simulink model "heli_sim"  (Simulink 7.7)
settings: Solver=ode4  SolverMode=SingleTasking  StartTime=0.0  StopTime=30  FixedStep=1/250  RelTol=1e-3
PostLoadFcn:
  | if exist('helicopter_sim.mat', 'file')
  |     load helicopter_sim.mat;
  | end
undefined symbols (not defined in the file or in its folder): alpha_IERA_IELA_IELA, in_cmd_final_value, in_CMD_ini, in_cmd_step_time, in_d_ini, in_omega_MR, in_omega_TR, in_outside_air_temp, in_pressure_altitude, in_xc_EOM_ini, R_IERA_RA_RA
libraries: simulink x4, UAVdesign_net x3
settings Model: Creator=Emanuel  LastModifiedBy=Emanuel  ExtModeLogAll=off
settings DataIOCC: LimitDataPoints=off  SaveFormat=StructureWithTime  SaveOutput=off  SignalLogging=off  SaveTime=off
settings OptimizationCC: InlineParams=on  SimCompilerOptimization=On
settings DebuggingCC: StrictBusMsg=Warning
settings HardwareCC: ProdIntDivRoundTo=Zero  ProdEndianess=LittleEndian  ProdHWDeviceType=Generic->32-bit x86 compatible
settings SFSimCC: SimParseCustomCode=off
settings RTWCC: RTWCompilerOptimization=On

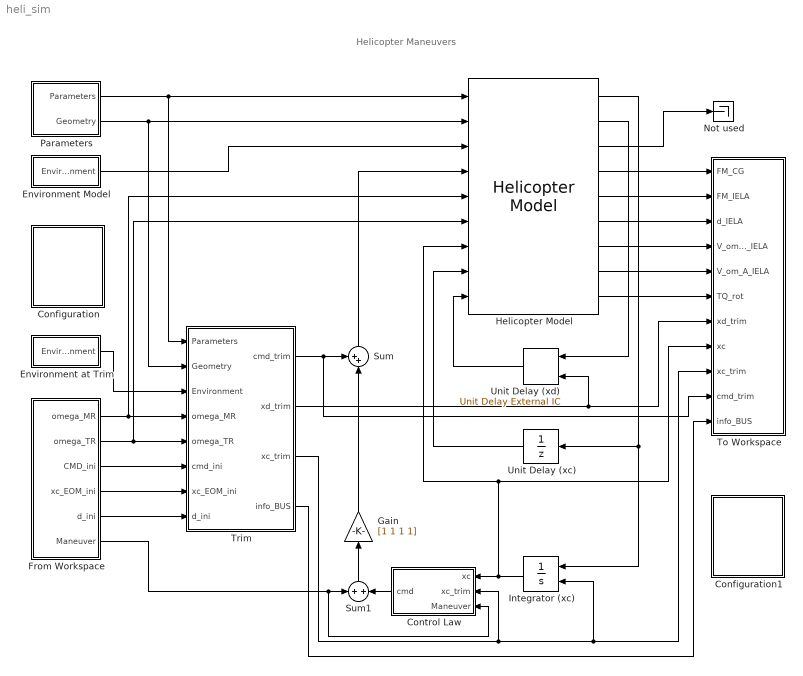
== system heli_sim ==
  note: Helicopter Maneuvers
  Configuration : Subsystem
      settings: OpenFcn=gui_HelicopterSim;
      mask Display: disp('Double-click\nto configure\nthe\nsimulation')
  Configuration1 : Subsystem
      settings: OpenFcn=graphs_Helicopter_sim;
      mask Display: disp('Double-click\nto display\nthe\ngraphs')
  Control Law : Subsystem
  Environment at Trim : Subsystem
  Environment Model : Subsystem
  From Workspace : Subsystem
  Gain : Gain  Gain=[1 1 1 1]
  Helicopter Model : UAVdesign_net/Vehicle Models/Helicopter Model  SystemSampleTime=-1
  Integrator (xc) : Integrator  InitialConditionSource=external  LimitOutput=on  UpperSaturationLimit="[1 1 1 1  1 1 1 1 100 100 100 inf inf inf pi/4 pi/4 pi/4 inf inf inf pi/4 pi/4 pi/4 pi/4 pi/4 pi/4]"  LowerSaturationLimit="-[1 1 1 1  1 1 1 1 100 100 100 inf inf inf pi/4 pi/4 pi/4 inf inf inf pi/4 pi/4 pi/4 pi/4 pi/4 pi/4]"
  Not used : Terminator
  Parameters : Subsystem
      mask init:
      | set_param(gcb, 'LinkStatus', 'none');
      settings: OpenFcn=gui_HelicopterParameters( 'Block', [get_param(gcb, 'Parent') '/' get_param(gcb, 'Name')]);
      mask Display:
      | port_label('output', 1, 'Parameters')
      | port_label('output', 2, 'Geometry')
  Sum : Sum  Inputs=++|
  Sum1 : Sum  Inputs=+|+
  To Workspace : Subsystem
  Trim : Subsystem
  Unit Delay (xc) : UnitDelay  X0=zeros(26,1)  SampleTime=1/250
  Unit Delay (xd) : simulink/Additional Math & Discrete/Additional Discrete/Unit Delay External IC  SystemSampleTime=-1  tsamp=1/250
  wires:
  Parameters/2(Geometry) -> Helicopter Model/2, Trim/2(Geometry)
  Parameters/1(Parameters) -> Helicopter Model/1, Trim/1(Parameters)
  Environment Model/1(Environment) -> Helicopter Model/3
  Unit Delay (xd)/1 -> Helicopter Model/9
  Helicopter Model/2 -> Unit Delay (xd)/1
  Trim/2(xd_trim) -> Unit Delay (xd)/2, To Workspace/7(xd_trim)
  Helicopter Model/1 -> Unit Delay (xc)/1, Integrator (xc)/1
  Unit Delay (xc)/1 -> Helicopter Model/8
  From Workspace/3(CMD_ini) -> Trim/6(cmd_ini)
  From Workspace/4(xc_EOM_ini) -> Trim/7(xc_EOM_ini)
  From Workspace/5(d_ini) -> Trim/8(d_ini)
  Integrator (xc)/1 -> Control Law/1(xc), Helicopter Model/7, To Workspace/8(xc)
  Trim/1(cmd_trim) -> Sum/1, To Workspace/10(cmd_trim)
  Sum/1 -> Helicopter Model/4
  Environment at Trim/1(Environment) -> Trim/3(Environment)
  From Workspace/2(omega_TR) -> Trim/5(omega_TR), Helicopter Model/6
  From Workspace/1(omega_MR) -> Trim/4(omega_MR), Helicopter Model/5
  Helicopter Model/3 -> Not used/1
  Helicopter Model/4 -> To Workspace/1(FM_CG)
  Helicopter Model/5 -> To Workspace/2(FM_IELA)
  Helicopter Model/6 -> To Workspace/3(d_IELA)
  Helicopter Model/7 -> To Workspace/4(V_om_W_IELA)
  Trim/4(info_BUS) -> To Workspace/11(info_BUS)
  Control Law/1(cmd) -> Sum1/2
  Trim/3(xc_trim) -> Control Law/2(xc_trim), Integrator (xc)/2, To Workspace/9(xc_trim)
  From Workspace/6(Maneuver) -> Sum1/1, Control Law/3(Maneuver)
  Helicopter Model/8 -> To Workspace/5(V_om_A_IELA)
  Helicopter Model/9 -> To Workspace/6(TQ_rot)
  Gain/1 -> Sum/2
  Sum1/1 -> Gain/1

== system heli_sim/Configuration ==

== system heli_sim/Configuration1 ==

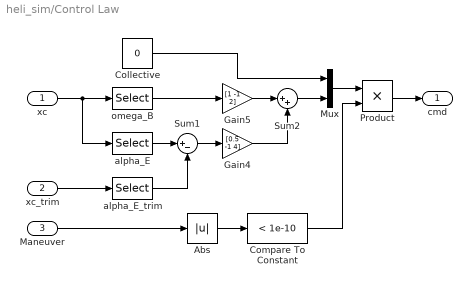
== system heli_sim/Control Law ==
  xc : Inport
  xc_trim : Inport  Port=2
  Maneuver : Inport  Port=3
  Abs : Abs
  Collective : Constant  Value=0
  Compare To Constant : simulink/Logic and Bit Operations/Compare To Constant  SystemSampleTime=-1  relop=<  const=1e-10  LogicOutDataTypeMode=boolean  ZeroCross=off
  Gain4 : Gain  Gain=[0.5 -1 4]
  Gain5 : Gain  Gain=[1 -1 2]
  Mux : Mux  Inputs=2
  Product : Product  RndMeth=Zero
  Sum1 : Sum  Inputs=|+-
  Sum2 : Sum  Inputs=|++
  alpha_E : Selector  InputPortWidth=26  IndexOptions=Index vector (dialog)  Indices=[18:20]  OutputSizes=1
  alpha_E_trim : Selector  InputPortWidth=26  IndexOptions=Index vector (dialog)  Indices=[18:20]  OutputSizes=1
  omega_B : Selector  InputPortWidth=26  IndexOptions=Index vector (dialog)  Indices=[15:17]  OutputSizes=1
  cmd : Outport
  wires:
  alpha_E_trim/1 -> Sum1/2
  alpha_E/1 -> Sum1/1
  Sum1/1 -> Gain4/1
  omega_B/1 -> Gain5/1
  xc/1 -> omega_B/1, alpha_E/1
  xc_trim/1 -> alpha_E_trim/1
  Gain5/1 -> Sum2/1
  Gain4/1 -> Sum2/2
  Sum2/1 -> Mux/2
  Collective/1 -> Mux/1
  Maneuver/1 -> Abs/1
  Mux/1 -> Product/1
  Product/1 -> cmd/1
  Compare To Constant/1 -> Product/2
  Abs/1 -> Compare To Constant/1

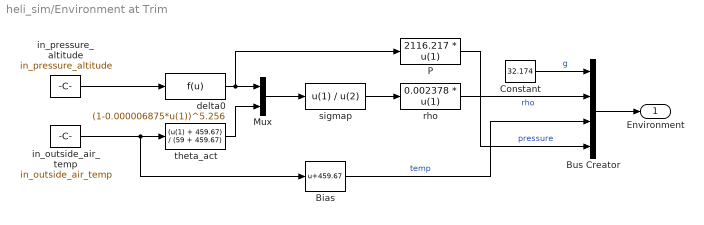
== system heli_sim/Environment at Trim ==
  Bias : Bias  Bias=459.67
  Bus Creator : BusCreator  OutDataTypeStr=Bus: Environment  NonVirtualBus=on
  Constant : Constant  Value=32.174
  Mux : Mux  Inputs=2
  P : Fcn  Expr=2116.217 * u(1)
  delta0 : Fcn  Expr=(1-0.000006875*u(1))^5.256
  in_outside_air_temp : Constant  Value=in_outside_air_temp
  in_pressure_altitude : Constant  Value=in_pressure_altitude
  rho : Fcn  Expr=0.002378 * u(1)
  sigmap : Fcn  Expr=u(1) / u(2)
  theta_act : Fcn  Expr=(u(1) + 459.67) / (59 + 459.67)
  Environment : Outport  OutDataTypeStr=Bus: Environment
  wires:
  sigmap/1 -> rho/1
  theta_act/1 -> Mux/2
  Mux/1 -> sigmap/1
  in_outside_air_temp/1 -> Bias/1, theta_act/1
  delta0/1 -> P/1, Mux/1
  in_pressure_altitude/1 -> delta0/1
  Bus Creator/1 -> Environment/1
  Constant/1 -> Bus Creator/1  "g"
  rho/1 -> Bus Creator/2  "rho"
  Bias/1 -> Bus Creator/3  "temp"
  P/1 -> Bus Creator/4  "pressure"

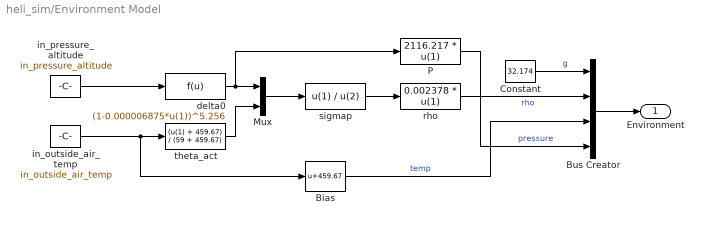
== system heli_sim/Environment Model ==
  Bias : Bias  Bias=459.67
  Bus Creator : BusCreator  OutDataTypeStr=Bus: Environment  NonVirtualBus=on
  Constant : Constant  Value=32.174
  Mux : Mux  Inputs=2
  P : Fcn  Expr=2116.217 * u(1)
  delta0 : Fcn  Expr=(1-0.000006875*u(1))^5.256
  in_outside_air_temp : Constant  Value=in_outside_air_temp
  in_pressure_altitude : Constant  Value=in_pressure_altitude
  rho : Fcn  Expr=0.002378 * u(1)
  sigmap : Fcn  Expr=u(1) / u(2)
  theta_act : Fcn  Expr=(u(1) + 459.67) / (59 + 459.67)
  Environment : Outport  OutDataTypeStr=Bus: Environment
  wires:
  P/1 -> Bus Creator/4  "pressure"
  Bias/1 -> Bus Creator/3  "temp"
  rho/1 -> Bus Creator/2  "rho"
  Constant/1 -> Bus Creator/1  "g"
  Bus Creator/1 -> Environment/1
  in_pressure_altitude/1 -> delta0/1
  delta0/1 -> Mux/1, P/1
  in_outside_air_temp/1 -> theta_act/1, Bias/1
  Mux/1 -> sigmap/1
  theta_act/1 -> Mux/2
  sigmap/1 -> rho/1

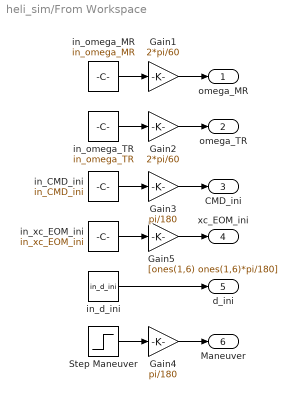
== system heli_sim/From Workspace ==
  Gain1 : Gain  Gain=2*pi/60
  Gain2 : Gain  Gain=2*pi/60
  Gain3 : Gain  Gain=pi/180
  Gain4 : Gain  Gain=pi/180
  Gain5 : Gain  Gain=[ones(1,6) ones(1,6)*pi/180]
  Step Maneuver : Step  Time=in_cmd_step_time  Before=[0 0 0 0]  After=in_cmd_final_value  SampleTime=0
  in_CMD_ini : Constant  Value=in_CMD_ini
  in_d_ini : Constant  Value=in_d_ini
  in_omega_MR : Constant  Value=in_omega_MR
  in_omega_TR : Constant  Value=in_omega_TR
  in_xc_EOM_ini : Constant  Value=in_xc_EOM_ini
  omega_MR : Outport
  omega_TR : Outport  Port=2
  CMD_ini : Outport  Port=3
  xc_EOM_ini : Outport  Port=4
  d_ini : Outport  Port=5
  Maneuver : Outport  Port=6
  wires:
  in_omega_MR/1 -> Gain1/1
  in_omega_TR/1 -> Gain2/1
  in_CMD_ini/1 -> Gain3/1
  in_xc_EOM_ini/1 -> Gain5/1
  in_d_ini/1 -> d_ini/1
  Gain4/1 -> Maneuver/1
  Step Maneuver/1 -> Gain4/1
  Gain1/1 -> omega_MR/1
  Gain2/1 -> omega_TR/1
  Gain3/1 -> CMD_ini/1
  Gain5/1 -> xc_EOM_ini/1

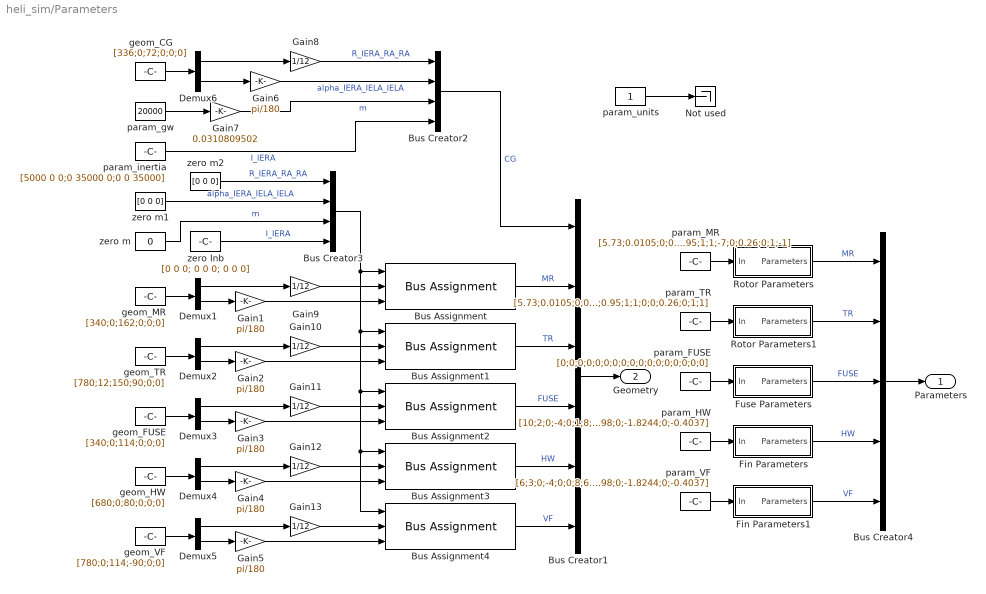
== system heli_sim/Parameters ==
  Bus Assignment{,1..4} (5 alike) : BusAssignment  AssignedSignals=R_IERA_RA_RA,alpha_IERA_IELA_IELA
  Bus Creator1 : BusCreator  Inputs=6
  Bus Creator2 : BusCreator  OutDataTypeStr=Bus: GeometryParameters
  Bus Creator3 : BusCreator  OutDataTypeStr=Bus: GeometryParameters
  Bus Creator4 : BusCreator  Inputs=5
  Demux{1..6} (6 alike) : Demux  Outputs=2
  Fin Parameters : Subsystem
  Fin Parameters1 : Subsystem
  Fuse Parameters : Subsystem
  Gain{1..6} (6 alike) : Gain  Gain=pi/180
  Gain{8..13} (6 alike) : Gain  Gain=1/12
  Gain7 : Gain  Gain=0.0310809502
  Not used : Terminator
  Rotor Parameters : Subsystem
  Rotor Parameters1 : Subsystem
  geom_CG : Constant  Value=[336;0;72;0;0;0]
  geom_FUSE : Constant  Value=[340;0;114;0;0;0]
  geom_HW : Constant  Value=[680;0;80;0;0;0]
  geom_MR : Constant  Value=[340;0;162;0;0;0]
  geom_TR : Constant  Value=[780;12;150;90;0;0]
  geom_VF : Constant  Value=[780;0;114;-90;0;0]
  param_FUSE : Constant  Value=[0;0;0;0;0;0;0;0;0;0;0;0;0;0;0;0;0]
  param_HW : Constant  Value=[10;2;0;-4;0;1;8;6.13;0.9682;1.8898;0;-1.8244;0;-0.4037]
  param_MR : Constant  Value=[5.73;0.0105;0;0.01325;0;-15;0;0;7;30;2.5;0.95;1;1;-7;0;0.26;0;1;-1]
  param_TR : Constant  Value=[5.73;0.0105;0;0.01325;0;-45;0;0;4;6.5;1.25;0.95;1;1;0;0;0.26;0;1;1]
  param_VF : Constant  Value=[6;3;0;-4;0;0;8;6.1311;0.9682;1.8898;0;-1.8244;0;-0.4037]
  param_gw : Constant  Value=20000
  param_inertia : Constant  Value=[5000 0 0;0 35000 0;0 0 35000]
  param_units : Constant
  zero Inb : Constant  Value=[0 0 0; 0 0 0; 0 0 0]
  zero m : Constant  Value=0
  zero m1 : Constant  Value=[0 0 0]
  zero m2 : Constant  Value=[0 0 0]
  Parameters : Outport
  Geometry : Outport  Port=2
  wires:
  Bus Creator2/1 -> Bus Creator1/1  "CG"
  Bus Assignment1/1 -> Bus Creator1/3  "TR"
  Bus Assignment2/1 -> Bus Creator1/4  "FUSE"
  Bus Assignment3/1 -> Bus Creator1/5  "HW"
  Bus Assignment4/1 -> Bus Creator1/6  "VF"
  Bus Creator1/1 -> Geometry/1
  Demux6/1 -> Gain8/1
  Demux6/2 -> Gain6/1
  param_gw/1 -> Gain7/1
  param_inertia/1 -> Bus Creator2/4  "I_IERA"
  Bus Assignment/1 -> Bus Creator1/2  "MR"
  Demux1/1 -> Gain9/1
  Demux1/2 -> Gain1/1
  geom_MR/1 -> Demux1/1
  Demux2/1 -> Gain10/1
  Demux2/2 -> Gain2/1
  geom_TR/1 -> Demux2/1
  Demux3/1 -> Gain11/1
  Demux3/2 -> Gain3/1
  geom_FUSE/1 -> Demux3/1
  Demux4/1 -> Gain12/1
  Demux4/2 -> Gain4/1
  geom_HW/1 -> Demux4/1
  Demux5/1 -> Gain13/1
  Demux5/2 -> Gain5/1
  geom_VF/1 -> Demux5/1
  geom_CG/1 -> Demux6/1
  Bus Creator3/1 -> Bus Assignment/1, Bus Assignment1/1, Bus Assignment2/1, Bus Assignment4/1, Bus Assignment3/1
  zero m/1 -> Bus Creator3/3  "m"
  zero m1/1 -> Bus Creator3/2  "alpha_IERA_IELA_IELA"
  zero Inb/1 -> Bus Creator3/4  "I_IERA"
  zero m2/1 -> Bus Creator3/1  "R_IERA_RA_RA"
  Bus Creator4/1 -> Parameters/1
  Rotor Parameters/1(Parameters) -> Bus Creator4/1  "MR"
  param_MR/1 -> Rotor Parameters/1(In)
  Rotor Parameters1/1(Parameters) -> Bus Creator4/2  "TR"
  param_TR/1 -> Rotor Parameters1/1(In)
  param_FUSE/1 -> Fuse Parameters/1(In)
  Fuse Parameters/1(Parameters) -> Bus Creator4/3  "FUSE"
  param_VF/1 -> Fin Parameters1/1(In)
  Fin Parameters1/1(Parameters) -> Bus Creator4/5  "VF"
  Fin Parameters/1(Parameters) -> Bus Creator4/4  "HW"
  param_HW/1 -> Fin Parameters/1(In)
  Gain1/1 -> Bus Assignment/3
  Gain2/1 -> Bus Assignment1/3
  Gain3/1 -> Bus Assignment2/3
  Gain4/1 -> Bus Assignment3/3
  Gain5/1 -> Bus Assignment4/3
  Gain6/1 -> Bus Creator2/2  "alpha_IERA_IELA_IELA"
  Gain7/1 -> Bus Creator2/3  "m"
  Gain8/1 -> Bus Creator2/1  "R_IERA_RA_RA"
  Gain9/1 -> Bus Assignment/2
  Gain10/1 -> Bus Assignment1/2
  Gain11/1 -> Bus Assignment2/2
  Gain12/1 -> Bus Assignment3/2
  Gain13/1 -> Bus Assignment4/2
  param_units/1 -> Not used/1

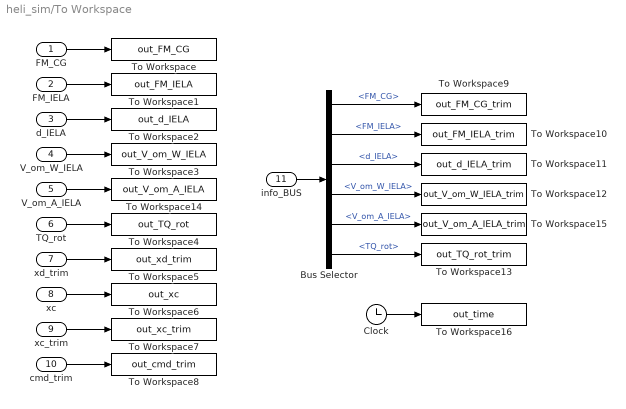
== system heli_sim/To Workspace ==
  FM_CG : Inport
  FM_IELA : Inport  Port=2
  d_IELA : Inport  Port=3
  V_om_W_IELA : Inport  Port=4
  V_om_A_IELA : Inport  Port=5
  TQ_rot : Inport  Port=6
  xd_trim : Inport  Port=7
  xc : Inport  Port=8
  xc_trim : Inport  Port=9
  cmd_trim : Inport  Port=10
  info_BUS : Inport  Port=11
  Bus Selector : BusSelector  OutputSignals=FM_CG,FM_IELA,d_IELA,V_om_W_IELA,V_om_A_IELA,TQ_rot
  Clock : Clock
  To Workspace : ToWorkspace  VariableName=out_FM_CG  SampleTime=-1  SaveFormat=Array
  To Workspace1 : ToWorkspace  VariableName=out_FM_IELA  SampleTime=-1  SaveFormat=Array
  To Workspace10 : ToWorkspace  VariableName=out_FM_IELA_trim  SampleTime=-1  SaveFormat=Array
      settings: MaxDataPoints=1
  To Workspace11 : ToWorkspace  VariableName=out_d_IELA_trim  SampleTime=-1  SaveFormat=Array
      settings: MaxDataPoints=1
  To Workspace12 : ToWorkspace  VariableName=out_V_om_W_IELA_trim  SampleTime=-1  SaveFormat=Array
      settings: MaxDataPoints=1
  To Workspace13 : ToWorkspace  VariableName=out_TQ_rot_trim  SampleTime=-1  SaveFormat=Array
      settings: MaxDataPoints=1
  To Workspace14 : ToWorkspace  VariableName=out_V_om_A_IELA  SampleTime=-1  SaveFormat=Array
  To Workspace15 : ToWorkspace  VariableName=out_V_om_A_IELA_trim  SampleTime=-1  SaveFormat=Array
      settings: MaxDataPoints=1
  To Workspace16 : ToWorkspace  VariableName=out_time  SampleTime=-1  SaveFormat=Array
  To Workspace2 : ToWorkspace  VariableName=out_d_IELA  SampleTime=-1  SaveFormat=Array
  To Workspace3 : ToWorkspace  VariableName=out_V_om_W_IELA  SampleTime=-1  SaveFormat=Array
  To Workspace4 : ToWorkspace  VariableName=out_TQ_rot  SampleTime=-1  SaveFormat=Array
  To Workspace5 : ToWorkspace  VariableName=out_xd_trim  SampleTime=-1  SaveFormat=Array
      settings: MaxDataPoints=1
  To Workspace6 : ToWorkspace  VariableName=out_xc  SampleTime=-1  SaveFormat=Array
  To Workspace7 : ToWorkspace  VariableName=out_xc_trim  SampleTime=-1  SaveFormat=Array
      settings: MaxDataPoints=1
  To Workspace8 : ToWorkspace  VariableName=out_cmd_trim  SampleTime=-1  SaveFormat=Array
      settings: MaxDataPoints=1
  To Workspace9 : ToWorkspace  VariableName=out_FM_CG_trim  SampleTime=-1  SaveFormat=Array
      settings: MaxDataPoints=1
  wires:
  FM_CG/1 -> To Workspace/1
  FM_IELA/1 -> To Workspace1/1
  d_IELA/1 -> To Workspace2/1
  V_om_W_IELA/1 -> To Workspace3/1
  TQ_rot/1 -> To Workspace4/1
  xd_trim/1 -> To Workspace5/1
  xc/1 -> To Workspace6/1
  xc_trim/1 -> To Workspace7/1
  cmd_trim/1 -> To Workspace8/1
  info_BUS/1 -> Bus Selector/1
  Bus Selector/1 -> To Workspace9/1  "<FM_CG>"
  Bus Selector/2 -> To Workspace10/1  "<FM_IELA>"
  Bus Selector/3 -> To Workspace11/1  "<d_IELA>"
  Bus Selector/4 -> To Workspace12/1  "<V_om_W_IELA>"
  Bus Selector/6 -> To Workspace13/1  "<TQ_rot>"
  V_om_A_IELA/1 -> To Workspace14/1
  Bus Selector/5 -> To Workspace15/1  "<V_om_A_IELA>"
  Clock/1 -> To Workspace16/1

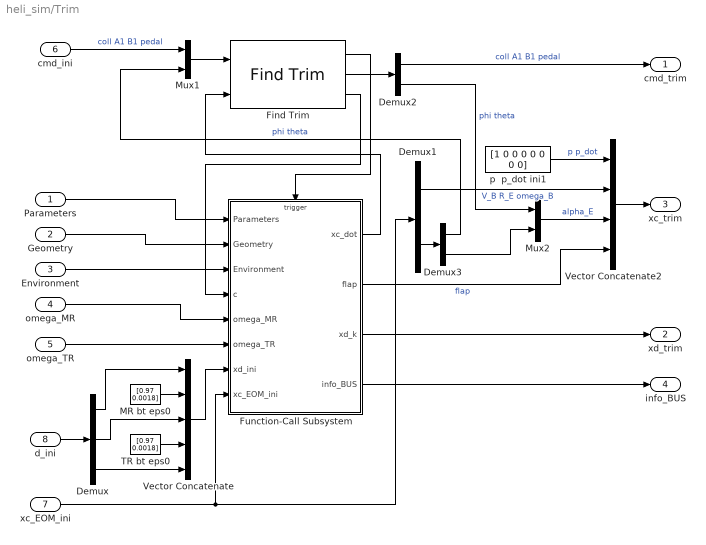
== system heli_sim/Trim ==
  Parameters : Inport
  Geometry : Inport  Port=2
  Environment : Inport  Port=3
  omega_MR : Inport  Port=4
  omega_TR : Inport  Port=5
  cmd_ini : Inport  Port=6
  xc_EOM_ini : Inport  Port=7
  d_ini : Inport  Port=8
  Demux : Demux  Outputs=[3 3 9]
  Demux1 : Demux  Outputs=[9 3]
  Demux2 : Demux  Outputs=[4 2]
  Demux3 : Demux  Outputs=[2 1]
  Find Trim : UAVdesign_net/Utilities/Numeric Perturbation/Find Trim  NumFInputs=6  NumFOutputs=6  RunOnce=on  SampleTime=-1
  Function-Call Subsystem : Subsystem  TreatAsAtomicUnit=on
  MR bt eps0 : Constant  Value=[0.97 0.0018]
  Mux1 : Mux  Inputs=2
  Mux2 : Mux  Inputs=2
  TR bt eps0 : Constant  Value=[0.97 0.0018]
  Vector Concatenate : Concatenate  NumInputs=5  Mode=Vector
  Vector Concatenate2 : Concatenate  NumInputs=4  Mode=Vector
  p  p_dot ini1 : Constant  Value="[1 0 0 0  0 0 0 0]"
  cmd_trim : Outport
  xd_trim : Outport  Port=2
  xc_trim : Outport  Port=3
  info_BUS : Outport  Port=4
  wires:
  Geometry/1 -> Function-Call Subsystem/2(Geometry)
  Parameters/1 -> Function-Call Subsystem/1(Parameters)
  omega_MR/1 -> Function-Call Subsystem/5(omega_MR)
  xc_EOM_ini/1 -> Function-Call Subsystem/8(xc_EOM_ini), Demux1/1
  omega_TR/1 -> Function-Call Subsystem/6(omega_TR)
  Find Trim/3 -> Function-Call Subsystem/4(c)
  Function-Call Subsystem/1(xc_dot) -> Find Trim/2
  Find Trim/1 -> Function-Call Subsystem/Trigger
  Function-Call Subsystem/3(xd_k) -> xd_trim/1
  d_ini/1 -> Demux/1
  Demux/1 -> Vector Concatenate/1
  MR bt eps0/1 -> Vector Concatenate/2
  Demux/2 -> Vector Concatenate/3
  TR bt eps0/1 -> Vector Concatenate/4
  Demux/3 -> Vector Concatenate/5
  Vector Concatenate/1 -> Function-Call Subsystem/7(xd_ini)
  Find Trim/2 -> Demux2/1
  Demux2/1 -> cmd_trim/1  "coll A1 B1 pedal"
  Mux1/1 -> Find Trim/1
  cmd_ini/1 -> Mux1/1  "coll A1 B1 pedal"
  Vector Concatenate2/1 -> xc_trim/1
  p  p_dot ini1/1 -> Vector Concatenate2/1  "p p_dot"
  Demux1/1 -> Vector Concatenate2/2  "V_B R_E omega_B"
  Mux2/1 -> Vector Concatenate2/3  "alpha_E"
  Function-Call Subsystem/2(flap) -> Vector Concatenate2/4  "flap"
  Demux3/2 -> Mux2/2
  Demux1/2 -> Demux3/1
  Demux2/2 -> Mux2/1  "phi theta"
  Demux3/1 -> Mux1/2  "phi theta"
  Environment/1 -> Function-Call Subsystem/3(Environment)
  Function-Call Subsystem/4(info_BUS) -> info_BUS/1

== system heli_sim/Parameters/Fin Parameters ==
  In : Inport
  Bus Creator : BusCreator  Inputs=14  OutDataTypeStr=Bus: FinParameters  NonVirtualBus=on
  Demux : Demux  Outputs=14
  Gain{,1..3} (4 alike) : Gain  Gain=pi/180
  Parameters : Outport  OutDataTypeStr=Bus: FinParameters
  wires:
  In/1 -> Demux/1
  Bus Creator/1 -> Parameters/1
  Demux/1 -> Bus Creator/1  "span"
  Demux/2 -> Bus Creator/2  "chord"
  Demux/3 -> Gain2/1
  Gain2/1 -> Bus Creator/3  "dihedral"
  Demux/4 -> Gain/1
  Gain/1 -> Bus Creator/4  "incid"
  Gain1/1 -> Bus Creator/5  "sweep"
  Demux/5 -> Gain1/1
  Demux/6 -> Bus Creator/6  "taper"
  Demux/7 -> Gain3/1
  Gain3/1 -> Bus Creator/7  "stall"
  Demux/8 -> Bus Creator/8  "a0"
  Demux/9 -> Bus Creator/9  "a1s2"
  Demux/10 -> Bus Creator/10  "cd0"
  Demux/11 -> Bus Creator/11  "cd1s1"
  Demux/12 -> Bus Creator/12  "cd2c1"
  Demux/13 -> Bus Creator/13  "cm0"
  Demux/14 -> Bus Creator/14  "cm1s1"

== system heli_sim/Parameters/Fin Parameters1 ==
  In : Inport
  Bus Creator : BusCreator  Inputs=14  OutDataTypeStr=Bus: FinParameters  NonVirtualBus=on
  Demux : Demux  Outputs=14
  Gain{,1..3} (4 alike) : Gain  Gain=pi/180
  Parameters : Outport  OutDataTypeStr=Bus: FinParameters
  wires:
  Demux/14 -> Bus Creator/14  "cm1s1"
  Demux/13 -> Bus Creator/13  "cm0"
  Demux/12 -> Bus Creator/12  "cd2c1"
  Demux/11 -> Bus Creator/11  "cd1s1"
  Demux/10 -> Bus Creator/10  "cd0"
  Demux/9 -> Bus Creator/9  "a1s2"
  Demux/8 -> Bus Creator/8  "a0"
  Gain3/1 -> Bus Creator/7  "stall"
  Demux/7 -> Gain3/1
  Demux/6 -> Bus Creator/6  "taper"
  Demux/5 -> Gain1/1
  Gain1/1 -> Bus Creator/5  "sweep"
  Gain/1 -> Bus Creator/4  "incid"
  Demux/4 -> Gain/1
  Gain2/1 -> Bus Creator/3  "dihedral"
  Demux/3 -> Gain2/1
  Demux/2 -> Bus Creator/2  "chord"
  Demux/1 -> Bus Creator/1  "span"
  Bus Creator/1 -> Parameters/1
  In/1 -> Demux/1

== system heli_sim/Parameters/Fuse Parameters ==
  In : Inport
  Bus Creator : BusCreator  Inputs=7  OutDataTypeStr=Bus: FuselageParameters  NonVirtualBus=on
  Demux : Demux  Outputs=17
  Vector Concatenate{,1..4} (5 alike) : Concatenate  NumInputs=3  Mode=Vector
  Parameters : Outport  OutDataTypeStr=Bus: FuselageParameters
  wires:
  Demux/1 -> Bus Creator/1  "carea"
  Bus Creator/1 -> Parameters/1
  In/1 -> Demux/1
  Demux/2 -> Bus Creator/2  "clen"
  Demux/3 -> Vector Concatenate/1
  Demux/4 -> Vector Concatenate/2
  Demux/5 -> Vector Concatenate/3
  Vector Concatenate/1 -> Bus Creator/3  "cx"
  Demux/6 -> Vector Concatenate1/1
  Demux/7 -> Vector Concatenate1/2
  Demux/8 -> Vector Concatenate1/3
  Vector Concatenate1/1 -> Bus Creator/4  "cy"
  Demux/9 -> Vector Concatenate2/1
  Demux/10 -> Vector Concatenate2/2
  Demux/11 -> Vector Concatenate2/3
  Vector Concatenate2/1 -> Bus Creator/5  "cz"
  Demux/12 -> Vector Concatenate3/1
  Demux/13 -> Vector Concatenate3/2
  Demux/14 -> Vector Concatenate3/3
  Demux/15 -> Vector Concatenate4/1
  Demux/16 -> Vector Concatenate4/2
  Demux/17 -> Vector Concatenate4/3
  Vector Concatenate3/1 -> Bus Creator/6  "cm"
  Vector Concatenate4/1 -> Bus Creator/7  "cn"

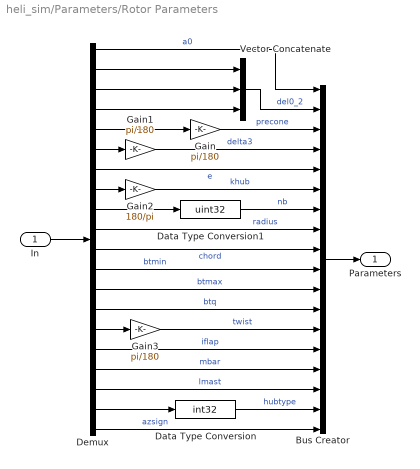
== system heli_sim/Parameters/Rotor Parameters ==
  In : Inport
  Bus Creator : BusCreator  Inputs=18  OutDataTypeStr=Bus: RotorParameters  NonVirtualBus=on
  Data Type Conversion : DataTypeConversion  OutDataTypeStr=int32  RndMeth=Nearest
  Data Type Conversion1 : DataTypeConversion  OutDataTypeStr=uint32  RndMeth=Nearest
  Demux : Demux  Outputs=20
  Gain : Gain  Gain=pi/180
  Gain1 : Gain  Gain=pi/180
  Gain2 : Gain  Gain=180/pi
  Gain3 : Gain  Gain=pi/180
  Vector Concatenate : Concatenate  NumInputs=3  Mode=Vector
  Parameters : Outport  OutDataTypeStr=Bus: RotorParameters
  wires:
  Demux/20 -> Bus Creator/18  "azsign"
  Demux/18 -> Bus Creator/16  "lmast"
  Demux/17 -> Bus Creator/15  "mbar"
  Demux/16 -> Bus Creator/14  "iflap"
  Demux/13 -> Bus Creator/11  "btmax"
  Demux/1 -> Bus Creator/1  "a0"
  Bus Creator/1 -> Parameters/1
  Demux/4 -> Vector Concatenate/3
  Demux/3 -> Vector Concatenate/2
  Demux/2 -> Vector Concatenate/1
  Vector Concatenate/1 -> Bus Creator/2  "del0_2"
  In/1 -> Demux/1
  Data Type Conversion/1 -> Bus Creator/17  "hubtype"
  Demux/19 -> Data Type Conversion/1
  Gain/1 -> Bus Creator/3  "precone"
  Gain1/1 -> Bus Creator/4  "delta3"
  Gain2/1 -> Bus Creator/6  "khub"
  Gain3/1 -> Bus Creator/13  "twist"
  Demux/5 -> Gain/1
  Demux/6 -> Gain1/1
  Demux/7 -> Bus Creator/5  "e"
  Demux/8 -> Gain2/1
  Data Type Conversion1/1 -> Bus Creator/7  "nb"
  Demux/9 -> Data Type Conversion1/1
  Demux/10 -> Bus Creator/8  "radius"
  Demux/11 -> Bus Creator/9  "chord"
  Demux/12 -> Bus Creator/10  "btmin"
  Demux/15 -> Gain3/1
  Demux/14 -> Bus Creator/12  "btq"

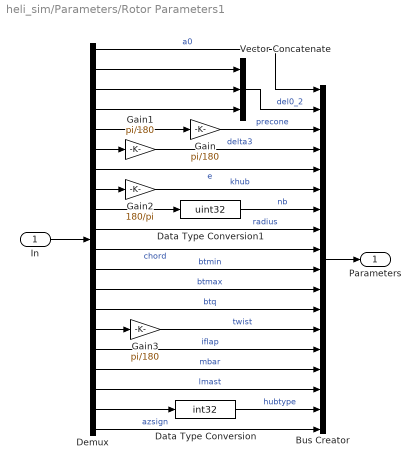
== system heli_sim/Parameters/Rotor Parameters1 ==
  In : Inport
  Bus Creator : BusCreator  Inputs=18  OutDataTypeStr=Bus: RotorParameters  NonVirtualBus=on
  Data Type Conversion : DataTypeConversion  OutDataTypeStr=int32  RndMeth=Nearest
  Data Type Conversion1 : DataTypeConversion  OutDataTypeStr=uint32  RndMeth=Nearest
  Demux : Demux  Outputs=20
  Gain : Gain  Gain=pi/180
  Gain1 : Gain  Gain=pi/180
  Gain2 : Gain  Gain=180/pi
  Gain3 : Gain  Gain=pi/180
  Vector Concatenate : Concatenate  NumInputs=3  Mode=Vector
  Parameters : Outport  OutDataTypeStr=Bus: RotorParameters
  wires:
  Demux/14 -> Bus Creator/12  "btq"
  Demux/15 -> Gain3/1
  Demux/12 -> Bus Creator/10  "btmin"
  Demux/11 -> Bus Creator/9  "chord"
  Demux/10 -> Bus Creator/8  "radius"
  Demux/9 -> Data Type Conversion1/1
  Data Type Conversion1/1 -> Bus Creator/7  "nb"
  Demux/8 -> Gain2/1
  Demux/7 -> Bus Creator/5  "e"
  Demux/6 -> Gain1/1
  Demux/5 -> Gain/1
  Gain3/1 -> Bus Creator/13  "twist"
  Gain2/1 -> Bus Creator/6  "khub"
  Gain1/1 -> Bus Creator/4  "delta3"
  Gain/1 -> Bus Creator/3  "precone"
  Demux/19 -> Data Type Conversion/1
  Data Type Conversion/1 -> Bus Creator/17  "hubtype"
  In/1 -> Demux/1
  Vector Concatenate/1 -> Bus Creator/2  "del0_2"
  Demux/2 -> Vector Concatenate/1
  Demux/3 -> Vector Concatenate/2
  Demux/4 -> Vector Concatenate/3
  Bus Creator/1 -> Parameters/1
  Demux/1 -> Bus Creator/1  "a0"
  Demux/13 -> Bus Creator/11  "btmax"
  Demux/16 -> Bus Creator/14  "iflap"
  Demux/17 -> Bus Creator/15  "mbar"
  Demux/18 -> Bus Creator/16  "lmast"
  Demux/20 -> Bus Creator/18  "azsign"

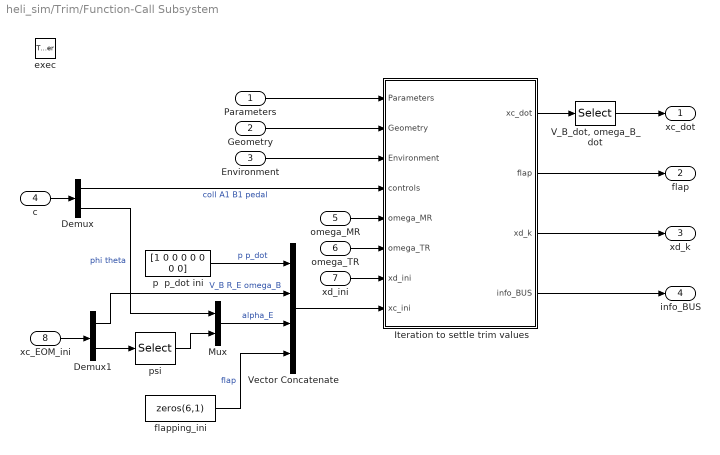
== system heli_sim/Trim/Function-Call Subsystem ==
  Parameters : Inport
  Geometry : Inport  Port=2
  Environment : Inport  Port=3
  c : Inport  Port=4
  omega_MR : Inport  Port=5
  omega_TR : Inport  Port=6
  xd_ini : Inport  Port=7
  xc_EOM_ini : Inport  Port=8
  exec : TriggerPort  TriggerType=function-call
  Demux : Demux  Outputs=[4 2]
  Demux1 : Demux  Outputs=[9 3]
  Iteration to settle trim values : Subsystem  TreatAsAtomicUnit=on
  Mux : Mux  Inputs=2
  "V_B_dot, omega_B_dot" : Selector  InputPortWidth=26  IndexOptions=Index vector (dialog)  Indices=[9:11 15:17]  OutputSizes=1
  Vector Concatenate : Concatenate  NumInputs=4  Mode=Vector
  flapping_ini : Constant  Value=zeros(6,1)
  p  p_dot ini : Constant  Value="[1 0 0 0  0 0 0 0]"
  psi : Selector  InputPortWidth=3  IndexOptions=Index vector (dialog)  Indices=[3]  OutputSizes=1
  xc_dot : Outport
  flap : Outport  Port=2
  xd_k : Outport  Port=3
  info_BUS : Outport  Port=4
  wires:
  Parameters/1 -> Iteration to settle trim values/1(Parameters)
  Geometry/1 -> Iteration to settle trim values/2(Geometry)
  omega_MR/1 -> Iteration to settle trim values/5(omega_MR)
  omega_TR/1 -> Iteration to settle trim values/6(omega_TR)
  c/1 -> Demux/1
  Demux/1 -> Iteration to settle trim values/4(controls)  "coll A1 B1 pedal"
  xd_ini/1 -> Iteration to settle trim values/7(xd_ini)
  Vector Concatenate/1 -> Iteration to settle trim values/8(xc_ini)
  p  p_dot ini/1 -> Vector Concatenate/1  "p p_dot"
  xc_EOM_ini/1 -> Demux1/1
  Demux1/1 -> Vector Concatenate/2  "V_B R_E omega_B"
  Mux/1 -> Vector Concatenate/3  "alpha_E"
  Demux/2 -> Mux/1  "phi theta"
  flapping_ini/1 -> Vector Concatenate/4  "flap"
  Iteration to settle trim values/1(xc_dot) -> "V_B_dot, omega_B_dot"/1
  "V_B_dot, omega_B_dot"/1 -> xc_dot/1
  Iteration to settle trim values/2(flap) -> flap/1
  Iteration to settle trim values/3(xd_k) -> xd_k/1
  psi/1 -> Mux/2
  Demux1/2 -> psi/1
  Environment/1 -> Iteration to settle trim values/3(Environment)
  Iteration to settle trim values/4(info_BUS) -> info_BUS/1

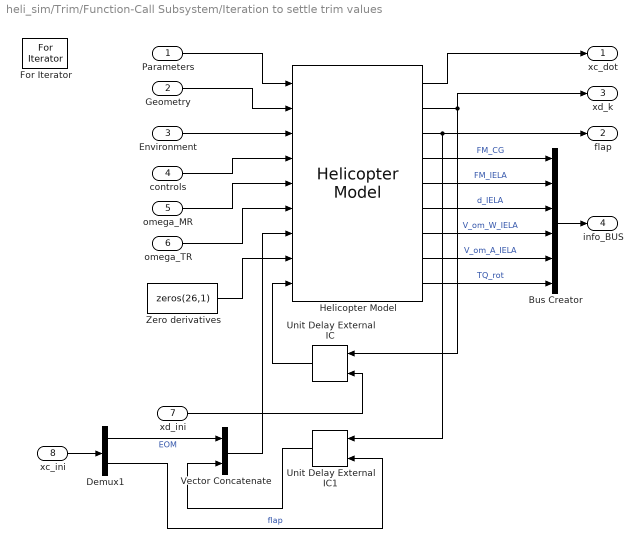
== system heli_sim/Trim/Function-Call Subsystem/Iteration to settle trim values ==
  Parameters : Inport
  Geometry : Inport  Port=2
  Environment : Inport  Port=3
  controls : Inport  Port=4
  omega_MR : Inport  Port=5
  omega_TR : Inport  Port=6
  xd_ini : Inport  Port=7
  xc_ini : Inport  Port=8
  Bus Creator : BusCreator  Inputs=6
  Demux1 : Demux  Outputs=[20 6]
  For Iterator : ForIterator  ResetStates=reset  IterationLimit=20  ShowIterationPort=off
  Helicopter Model : UAVdesign_net/Vehicle Models/Helicopter Model  SystemSampleTime=-1
  Unit Delay External IC : simulink/Additional Math & Discrete/Additional Discrete/Unit Delay External IC  SystemSampleTime=-1  tsamp=-1
  Unit Delay External IC1 : simulink/Additional Math & Discrete/Additional Discrete/Unit Delay External IC  SystemSampleTime=-1  tsamp=-1
  Vector Concatenate : Concatenate  Mode=Vector
  Zero derivatives : Constant  Value=zeros(26,1)
  xc_dot : Outport
  flap : Outport  Port=2
  xd_k : Outport  Port=3
  info_BUS : Outport  Port=4
  wires:
  Unit Delay External IC1/1 -> Vector Concatenate/2
  Demux1/2 -> Unit Delay External IC1/2  "flap"
  Demux1/1 -> Vector Concatenate/1  "EOM"
  Vector Concatenate/1 -> Helicopter Model/7
  xc_ini/1 -> Demux1/1
  Helicopter Model/3 -> Unit Delay External IC1/1, flap/1
  Zero derivatives/1 -> Helicopter Model/8
  xd_ini/1 -> Unit Delay External IC/2
  omega_TR/1 -> Helicopter Model/6
  omega_MR/1 -> Helicopter Model/5
  controls/1 -> Helicopter Model/4
  Environment/1 -> Helicopter Model/3
  Geometry/1 -> Helicopter Model/2
  Parameters/1 -> Helicopter Model/1
  Helicopter Model/1 -> xc_dot/1
  Helicopter Model/2 -> Unit Delay External IC/1, xd_k/1
  Unit Delay External IC/1 -> Helicopter Model/9
  Bus Creator/1 -> info_BUS/1
  Helicopter Model/4 -> Bus Creator/1  "FM_CG"
  Helicopter Model/5 -> Bus Creator/2  "FM_IELA"
  Helicopter Model/6 -> Bus Creator/3  "d_IELA"
  Helicopter Model/7 -> Bus Creator/4  "V_om_W_IELA"
  Helicopter Model/9 -> Bus Creator/6  "TQ_rot"
  Helicopter Model/8 -> Bus Creator/5  "V_om_A_IELA"
